simulink model "Lab3_Crazyflie_VirtualTemplate2023"  (R2022b)
settings: Solver=FixedStepAuto  StartTime=0.0  StopTime=inf  MaxStep=0.1  RelTol=1e-3  EnableMultiTasking=on
PreLoadFcn:
  | % load parameters of the default quadrotor
  | disp('Quadrotor parameters loaded by PreLoadFcn')
  | mdl_quadrotor
undefined symbols (not defined in the file or in its folder): Angular, Linear, rot2
libraries: robotlib x4
settings Model: Creator=corkep  LastModifiedBy=marios
settings SolverCC: AlgebraicLoopSolver=TrustRegion
settings DataIOCC: LimitDataPoints=on  ReturnWorkspaceOutputs=off
settings OptimizationCC: EnhancedBackFolding=on  PassReuseOutputArgsAs=Individual arguments  ExpressionDepthLimit=2147483647  ZeroExternalMemoryAtStartup=off  ZeroInternalMemoryAtStartup=off  MaxStackSize=64  OptimizeBlockOrder=speed  DifferentSizesBufferReuse=on  OptimizationCustomize=off  EfficientTunableParamExpr=on
settings DebuggingCC: UnderspecifiedInitializationDetection=Classic  MergeDetectMultiDrivingBlocksExec=none  SolverPrmCheckMsg=warning  ParameterTunabilityLossMsg=error  UnconnectedInputMsg=warning  UnconnectedOutputMsg=warning  UnconnectedLineMsg=warning  AllowSymbolicDim=off  StateNameClashWarn=warning  SFUnexpectedBacktrackingDiag=warning  SFNoUnconditionalDefaultTransitionDiag=warning  SFExecutionAtInitializationDiag=none  SFMachineParentedDataDiag=warning  ArithmeticOperatorsInVariantConditions=warning
settings HardwareCC: ProdBitPerPointer=32  ProdBitPerSizeT=32  ProdBitPerPtrDiffT=32  ProdLargestAtomicFloat=None  ProdIntDivRoundTo=Undefined  ProdEndianess=Unspecified  ProdWordSize=32  ProdHWDeviceType=Generic->Unspecified (assume 32-bit Generic)  UseEmbeddedCoderFeatures=off
settings ModelReferenceCC: EnableRefExpFcnMdlSchedulingChecks=on  PropagateSignalLabelsOutOfModel=off
settings SFSimCC: SimUseLocalCustomCode=off  MATLABDynamicMemAlloc=off  CustomCodeUndefinedFunction=UseInterfaceOnly
settings RTWCC: Description=Embedded Coder  SystemTargetFile=ert.tlc  HardwareBoard=Robot Operating System (ROS)  TLCOptions="-aInlineSetEventsForThisBaseRateFcn=TLC_FALSE -aSuppressMultiTaskScheduler=TLC_FALSE  -aRateBasedStepFcn=0"  TemplateMakefile=ert_default_tmf  RTWUseLocalCustomCode=off  Toolchain=Catkin  TargetLang=C++
settings CodeAppCC: ForceParamTrailComments=on  IgnoreCustomStorageClasses=off  OperatorAnnotations=on  SimulinkDataObjDesc=on  SFDataObjDesc=on  InsertBlockDesc=on
settings ERTTargetCC: SupportNonInlinedSFcns=on
settings ConfigComp: CovMetricSettings=dw  CovSaveCumulativeToWorkspaceVar=on  CovSaveSingleToWorkspaceVar=on  CovExternalEMLEnable=off  CovSFcnEnable=off

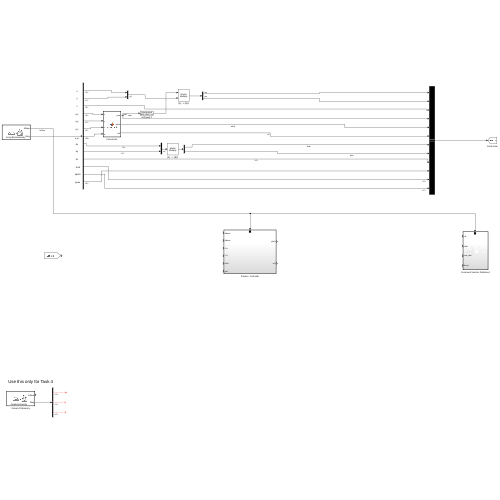
[thumbnail: Simulink's stored preview of the top-level diagram]
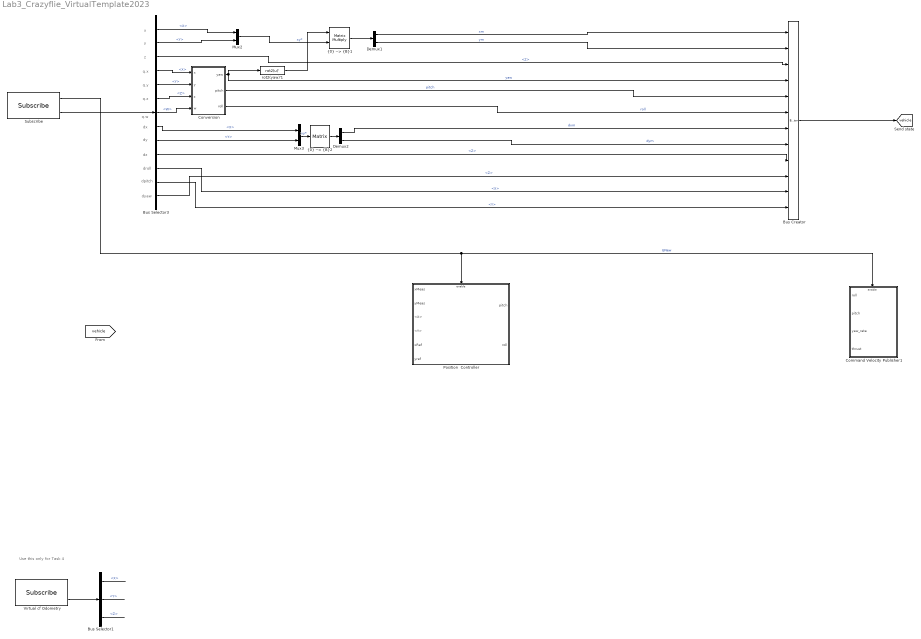
== system Lab3_Crazyflie_VirtualTemplate2023 ==
  note: Use this only for Task 4
  note: dyaw
  note: dpitch
  note: droll
  note: dz
  note: dy
  note: dx
  note: x
  note: y
  note: z
  note: q.x
  note: q.y
  note: q.z
  note: q.w
  Bus Creator : BusCreator  Inputs=12
  Bus Selector1 : BusSelector  OutputSignals=Pose.Pose.Position.X,Pose.Pose.Position.Y,Pose.Pose.Position.Z
  Bus Selector3 : BusSelector  OutputSignals=Pose.Pose.Position.X,Pose.Pose.Position.Y,Pose.Pose.Position.Z,Pose.Pose.Orientation.X,Pose.Pose.Orientation.Y,Pose.Pose.Orientation.Z,Pose.Pose.Orientation.W,Twist.Twist.Linear.X,Twist.Twist.Linear.Y,Twist.Twist.Linear.Z,Twist.Twist.Angular.X,Twist.Twist.Angular.Y,Twist.Twist.Angular.Z
  Command Velocity Publisher1 : Subsystem
  Conversion : MATLAB Function  TreatAsAtomicUnit=on
  Demux1 : Demux  Outputs=2
  Demux2 : Demux  Outputs=2
  Mux2 : Mux  Inputs=2
  Mux3 : Mux  Inputs=2
  Position  Controller : Subsystem
  Subscribe : robotlib/Subscribe  topicSource=Select from ROS network  topic=/crazyflie2/odometry  messageType=nav_msgs/Odometry  SampleTime=-1  legacyBusStruct=off  messageQueueLength=51
  Virtual cf Odometry : robotlib/Subscribe  topicSource=Specify your own  topic=/leader/odometry  messageType=nav_msgs/Odometry  SampleTime=-1  legacyBusStruct=off  messageQueueLength=51
  rot2(yaw)'1 : MATLABFcn  MATLABFcn=rot2(u)'  OutputDimensions=[2 2]  Output1D=off
  "{0} --> {B}1" : Product  Multiplication=Matrix(*)  RndMeth=Zero
  "{0} --> {B}2" : Product  Inputs=1  Multiplication=Matrix(*)  RndMeth=Zero
  tag scope: vehicle=global
  wires:
  Bus Selector3/11 -> Bus Creator/11  "<X>"
  Bus Selector3/13 -> Bus Creator/10  "<Z>"
  Conversion/1(yaw) -> rot2(yaw)'1/1, Bus Creator/4  "yaw"
  Bus Selector3/10 -> Bus Creator/9  "<Z>"
  Bus Selector3/9 -> Mux3/2  "<Y>"
  Bus Selector3/8 -> Mux3/1  "<X>"
  Conversion/2(pitch) -> Bus Creator/5  "pitch"
  Bus Creator/1 -> [vehicle]
  Bus Selector3/12 -> Bus Creator/12  "<Y>"
  Conversion/3(roll) -> Bus Creator/6  "roll"
  Subscribe/2 -> Bus Selector3/1
  Bus Selector3/4 -> Conversion/1(x)  "<X>"
  Bus Selector3/5 -> Conversion/2(y)  "<Y>"
  Bus Selector3/6 -> Conversion/3(z)  "<Z>"
  Bus Selector3/7 -> Conversion/4(w)  "<W>"
  Subscribe/1 -> Command Velocity Publisher1/Enable, Position  Controller/Enable  "IsNew"
  Mux2/1 -> "{0} --> {B}1"/2  "xy*"
  "{0} --> {B}1"/1 -> Demux1/1
  "{0} --> {B}2"/1 -> Demux2/1
  Demux1/1 -> Bus Creator/1  "xm"
  Demux1/2 -> Bus Creator/2  "ym"
  Bus Selector3/1 -> Mux2/1  "<X>"
  Bus Selector3/2 -> Mux2/2  "<Y>"
  Demux2/1 -> Bus Creator/7  "dxm"
  Demux2/2 -> Bus Creator/8  "dym"
  Mux3/1 -> "{0} --> {B}2"/1  "xy*"
  Bus Selector3/3 -> Bus Creator/3  "<Z>"
  rot2(yaw)'1/1 -> "{0} --> {B}1"/1
  Virtual cf Odometry/2 -> Bus Selector1/1
  Bus Selector1/1 -> ?  "<X>"
  Bus Selector1/2 -> ?  "<Y>"
  Bus Selector1/3 -> ?  "<Z>"

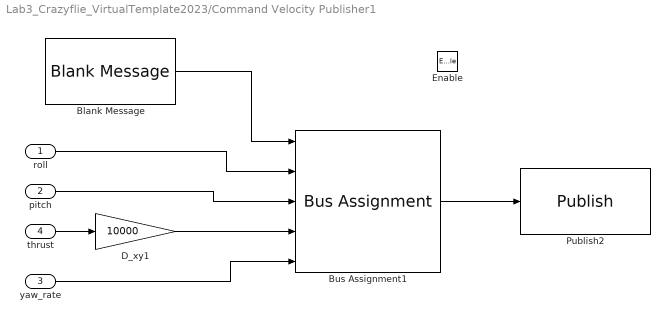
== system Lab3_Crazyflie_VirtualTemplate2023/Command Velocity Publisher1 ==
  roll : Inport
  pitch : Inport  Port=2
  yaw_rate : Inport  Port=3
  thrust : Inport  Port=4
  Enable : EnablePort
  Blank Message : robotlib/Blank Message  messageClass=Message  entityType=geometry_msgs/Twist  messageType=geometry_msgs/Twist  SampleTime=inf  legacyBusStruct=off
  Bus Assignment1 : BusAssignment  DialogController=Simulink.DDGSource_BusAssignment  AssignedSignals=Linear.X,Linear.Y,Linear.Z,Angular.Z
  D_xy1 : Gain  Gain=10000
  Publish2 : robotlib/Publish  topicSource=Select from ROS network  topic=/crazyflie2/cmd_vel  messageType=geometry_msgs/Twist  legacyBusStruct=off  messageQueueLength=105
  wires:
  Bus Assignment1/1 -> Publish2/1
  Blank Message/1 -> Bus Assignment1/1
  roll/1 -> Bus Assignment1/2
  pitch/1 -> Bus Assignment1/3
  thrust/1 -> D_xy1/1
  yaw_rate/1 -> Bus Assignment1/5
  D_xy1/1 -> Bus Assignment1/4

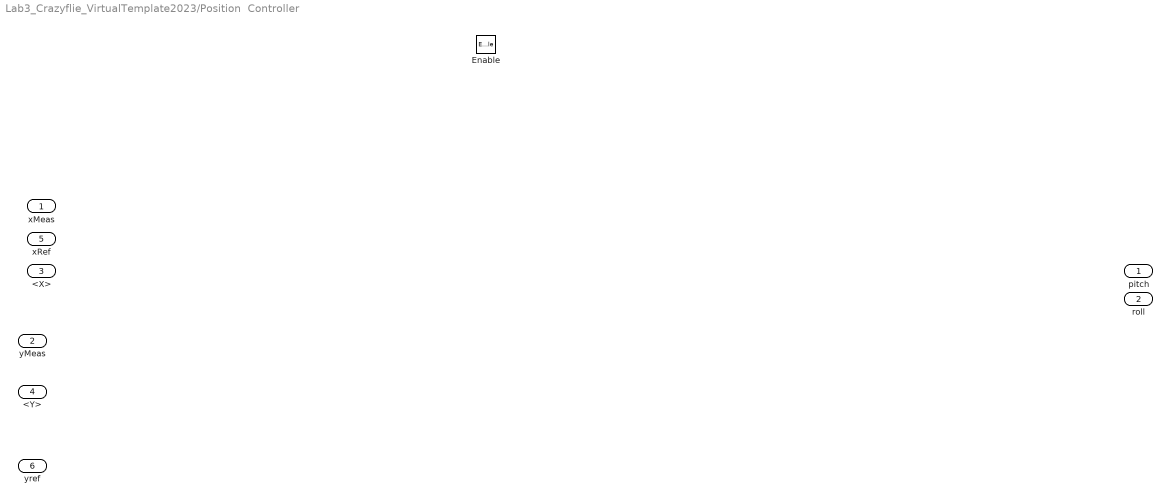
== system Lab3_Crazyflie_VirtualTemplate2023/Position  Controller ==
  xMeas : Inport
  yMeas : Inport  Port=2
  <X> : Inport  Port=3
  <Y> : Inport  Port=4
  xRef : Inport  Port=5
  yref : Inport  Port=6
  Enable : EnablePort
  pitch : Outport
  roll : Outport  Port=2

== matlab function Lab3_Crazyflie_VirtualTemplate2023/Conversion ==
  data: yaw output; x input; y input; z input; w input; pitch output; roll output
function [yaw,pitch,roll]  = quat2eul(x,y,z,w)
%#codegen

% Convert the quaternion to a yaw angle (zyx euler angle)
eul = quat2eul([w,x,y,z]);
yaw = eul(1);
roll = eul(3);
pitch = eul(2);

end
